simulink model "TEST1231"  (R2021a)
settings: Solver=VariableStepAuto  StartTime=0.0  StopTime=10.0  RelTol=1e-3
values from neighbouring files (symbols this model uses):
  phi0 = 0    [test.m]
  Rmin = 6    [Copy_of_main.m]    (also in parall.m)
  x0 = -8.5    [paralle.m]    (also in test.m = 9; verit.m = -3.7)
  y0 = -4    [paralle.m]    (also in test.m = 3; verit.m = -6.5)
libraries: dspstat3 x2
settings Model: Creator=6000022764  LastModifiedBy=6000022764

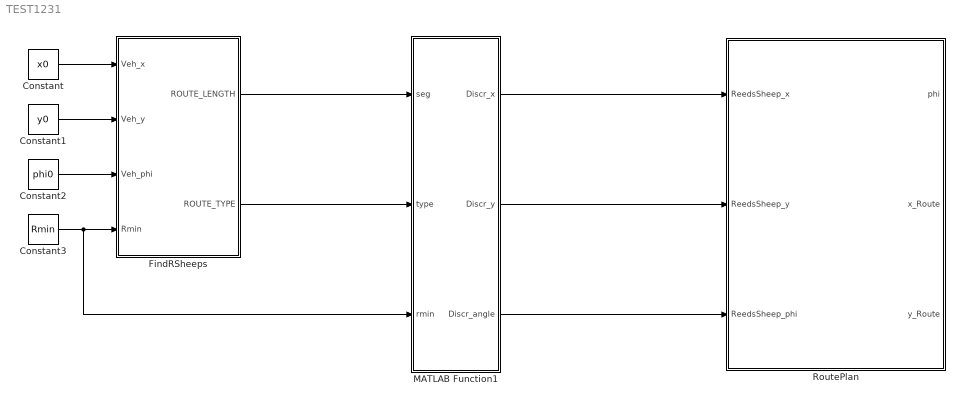
== system TEST1231 ==
  Constant : Constant  Value=x0
  Constant1 : Constant  Value=y0
  Constant2 : Constant  Value=phi0
  Constant3 : Constant  Value=Rmin
  FindRSheeps : Subsystem  Description=查找RS路径
      settings: AttributesFormatString=%<Description>
  MATLAB Function1 : MATLAB Function  TreatAsAtomicUnit=on
  RoutePlan : Subsystem  Description=B样条曲线
      settings: AttributesFormatString=%<Description>
  wires:
  Constant/1 -> FindRSheeps/1(Veh_x)
  Constant1/1 -> FindRSheeps/2(Veh_y)
  Constant3/1 -> MATLAB Function1/3(rmin), FindRSheeps/4(Rmin)
  Constant2/1 -> FindRSheeps/3(Veh_phi)
  FindRSheeps/1(ROUTE_LENGTH) -> MATLAB Function1/1(seg)
  FindRSheeps/2(ROUTE_TYPE) -> MATLAB Function1/2(type)
  MATLAB Function1/1(Discr_x) -> RoutePlan/1(ReedsSheep_x)
  MATLAB Function1/2(Discr_y) -> RoutePlan/2(ReedsSheep_y)
  MATLAB Function1/3(Discr_angle) -> RoutePlan/3(ReedsSheep_phi)

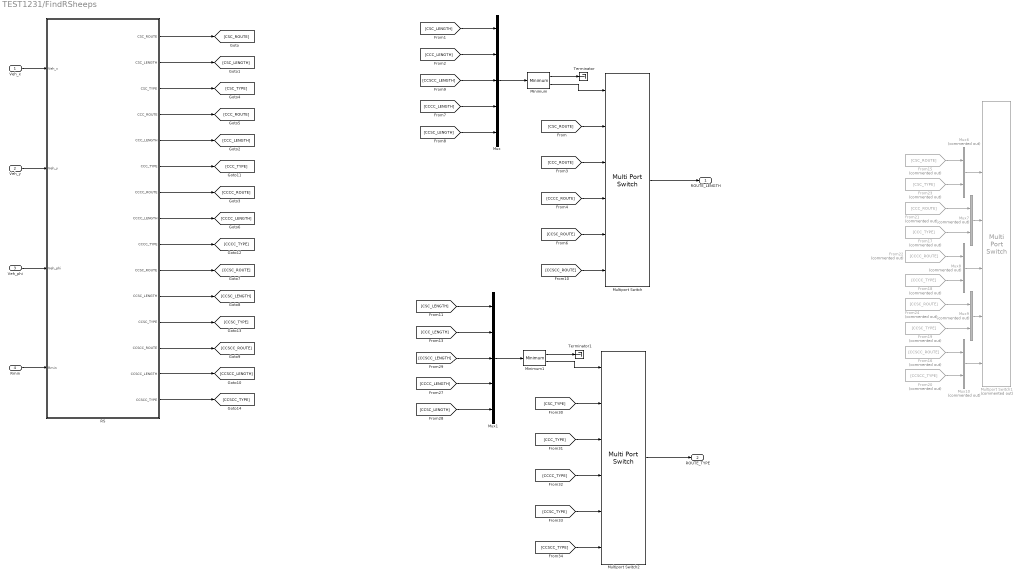
== system TEST1231/FindRSheeps ==
  Veh_x : Inport
  Veh_y : Inport  Port=2
  Veh_phi : Inport  Port=3
  Rmin : Inport  Port=4
  From15 : From  Commented=on  GotoTag=CSC_ROUTE
  From16 : From  Commented=on  GotoTag=CCSCC_ROUTE
  From17 : From  Commented=on  GotoTag=CCC_TYPE
  From18 : From  Commented=on  GotoTag=CCCC_TYPE
  From19 : From  Commented=on  GotoTag=CCSC_TYPE
  From20 : From  Commented=on  GotoTag=CCSCC_TYPE
  From21 : From  Commented=on  GotoTag=CCC_ROUTE
  From22 : From  Commented=on  GotoTag=CCCC_ROUTE
  From23 : From  Commented=on  GotoTag=CSC_TYPE
  From24 : From  Commented=on  GotoTag=CCSC_ROUTE
  Minimum : dspstat3/Minimum  operation=minimum  fcn=Value and Index  indexBase=One  operateOver=Each column  Dimension=1  InputProcessing=Columns as channels (frame based)  reset=None  roiEnable=off  roiType=Rectangles  roiPortion=Entire ROI  roiOutput=Individual statistics for each ROI  roiFlag=off  roundingMode=Floor  overflowMode=off
      settings: SourceProductBaseCode=DS
  Minimum1 : dspstat3/Minimum  operation=minimum  fcn=Value and Index  indexBase=One  operateOver=Each column  Dimension=1  InputProcessing=Columns as channels (frame based)  reset=None  roiEnable=off  roiType=Rectangles  roiPortion=Entire ROI  roiOutput=Individual statistics for each ROI  roiFlag=off  roundingMode=Floor  overflowMode=off
      settings: SourceProductBaseCode=DS
  Multiport Switch : MultiPortSwitch  Inputs=5
  Multiport Switch1 : MultiPortSwitch  Commented=on  Inputs=5
  Multiport Switch2 : MultiPortSwitch  Inputs=5
  Mux : Mux  Inputs=5
  Mux1 : Mux  Inputs=5
  Mux{6..10} (5 alike) : Mux  Commented=on  Inputs=2
  RS : Subsystem  Description=RS_word
      settings: AttributesFormatString=%<Description>
  Terminator : Terminator
  Terminator1 : Terminator
  ROUTE_LENGTH : Outport
  ROUTE_TYPE : Outport  Port=2
  wires:
  Minimum/1 -> Terminator/1
  [CCSCC_ROUTE] -> Multiport Switch/6
  [CCSC_ROUTE] -> Multiport Switch/5
  [CCC_ROUTE] -> Multiport Switch/3
  [CCCC_ROUTE] -> Multiport Switch/4
  RS/15(CCSCC_TYPE) -> [CCSCC_TYPE]
  RS/12(CCSC_TYPE) -> [CCSC_TYPE]
  RS/9(CCCC_TYPE) -> [CCCC_TYPE]
  RS/6(CCC_TYPE) -> [CCC_TYPE]
  [CSC_ROUTE] -> Multiport Switch/2
  RS/3(CSC_TYPE) -> [CSC_TYPE]
  Multiport Switch/1 -> ROUTE_LENGTH/1
  [CCSCC_LENGTH] -> Mux/3
  [CCSC_LENGTH] -> Mux/5
  [CCCC_LENGTH] -> Mux/4
  RS/14(CCSCC_LENGTH) -> [CCSCC_LENGTH]
  RS/13(CCSCC_ROUTE) -> [CCSCC_ROUTE]
  RS/11(CCSC_LENGTH) -> [CCSC_LENGTH]
  RS/10(CCSC_ROUTE) -> [CCSC_ROUTE]
  RS/8(CCCC_LENGTH) -> [CCCC_LENGTH]
  RS/7(CCCC_ROUTE) -> [CCCC_ROUTE]
  RS/5(CCC_LENGTH) -> [CCC_LENGTH]
  RS/4(CCC_ROUTE) -> [CCC_ROUTE]
  RS/2(CSC_LENGTH) -> [CSC_LENGTH]
  RS/1(CSC_ROUTE) -> [CSC_ROUTE]
  Rmin/1 -> RS/4(Rmin)
  Veh_phi/1 -> RS/3(Veh_phi)
  Veh_y/1 -> RS/2(Veh_y)
  Veh_x/1 -> RS/1(Veh_x)
  [CCC_LENGTH] -> Mux/2
  [CSC_LENGTH] -> Mux/1
  Mux/1 -> Minimum/1
  Minimum/2 -> Multiport Switch/1
  From15/1 -> Mux6/1
  From23/1 -> Mux6/2
  Mux6/1 -> Multiport Switch1/2
  From21/1 -> Mux7/1
  From17/1 -> Mux7/2
  From22/1 -> Mux8/1
  From18/1 -> Mux8/2
  From24/1 -> Mux9/1
  From19/1 -> Mux9/2
  From16/1 -> Mux10/1
  From20/1 -> Mux10/2
  Mux8/1 -> Multiport Switch1/4
  Mux7/1 -> Multiport Switch1/3
  Mux9/1 -> Multiport Switch1/5
  Mux10/1 -> Multiport Switch1/6
  Minimum1/2 -> Multiport Switch2/1
  Mux1/1 -> Minimum1/1
  [CSC_LENGTH] -> Mux1/1
  [CCC_LENGTH] -> Mux1/2
  [CCCC_LENGTH] -> Mux1/4
  [CCSC_LENGTH] -> Mux1/5
  [CCSCC_LENGTH] -> Mux1/3
  Multiport Switch2/1 -> ROUTE_TYPE/1
  [CSC_TYPE] -> Multiport Switch2/2
  [CCCC_TYPE] -> Multiport Switch2/4
  [CCC_TYPE] -> Multiport Switch2/3
  [CCSC_TYPE] -> Multiport Switch2/5
  [CCSCC_TYPE] -> Multiport Switch2/6
  Minimum1/1 -> Terminator1/1

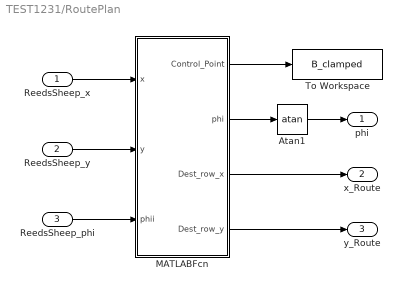
== system TEST1231/RoutePlan ==
  ReedsSheep_x : Inport
  ReedsSheep_y : Inport  Port=2
  ReedsSheep_phi : Inport  Port=3
  Atan1 : Trigonometry  Operator=atan
  MATLABFcn : MATLAB Function  Description=5次B样条开Clamped  TreatAsAtomicUnit=on
      settings: AttributesFormatString=%<Description>
  To Workspace : ToWorkspace  VariableName=B_clamped  SampleTime=-1
  phi : Outport  InitialOutput=0
  x_Route : Outport  Port=2  InitialOutput=9
  y_Route : Outport  Port=3  InitialOutput=3
  wires:
  MATLABFcn/1(Control_Point) -> To Workspace/1
  MATLABFcn/2(phi) -> Atan1/1
  Atan1/1 -> phi/1
  MATLABFcn/3(Dest_row_x) -> x_Route/1
  MATLABFcn/4(Dest_row_y) -> y_Route/1
  ReedsSheep_x/1 -> MATLABFcn/1(x)
  ReedsSheep_y/1 -> MATLABFcn/2(y)
  ReedsSheep_phi/1 -> MATLABFcn/3(phii)

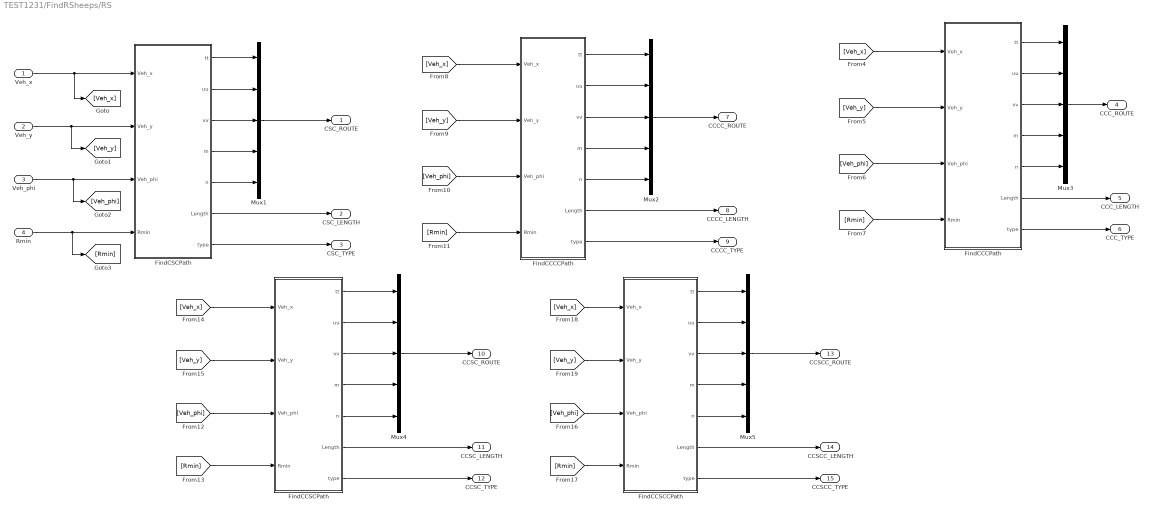
== system TEST1231/FindRSheeps/RS ==
  Veh_x : Inport
  Veh_y : Inport  Port=2
  Veh_phi : Inport  Port=3
  Rmin : Inport  Port=4
  FindCCCCPath : Stateflow chart  Description=查找CCCC路径  TreatAsAtomicUnit=on
      settings: AttributesFormatString=%<Description>  RTWSystemCode=Inline
  FindCCCPath : Stateflow chart  Description=查找CCC路径  TreatAsAtomicUnit=on
      settings: AttributesFormatString=%<Description>  RTWSystemCode=Inline
  FindCCSCCPath : Stateflow chart  Description=查找CCSCC路径  TreatAsAtomicUnit=on
      settings: AttributesFormatString=%<Description>  RTWSystemCode=Inline
  FindCCSCPath : Stateflow chart  Description=查找CCSC路径  TreatAsAtomicUnit=on
      settings: AttributesFormatString=%<Description>  RTWSystemCode=Inline
  FindCSCPath : Stateflow chart  Description=查找CSC路径  TreatAsAtomicUnit=on
      settings: AttributesFormatString=%<Description>  RTWSystemCode=Inline
  Mux{1..5} (5 alike) : Mux  Inputs=5
  CSC_ROUTE : Outport
  CSC_LENGTH : Outport  Port=2
  CSC_TYPE : Outport  Port=3
  CCC_ROUTE : Outport  Port=4
  CCC_LENGTH : Outport  Port=5
  CCC_TYPE : Outport  Port=6
  CCCC_ROUTE : Outport  Port=7
  CCCC_LENGTH : Outport  Port=8
  CCCC_TYPE : Outport  Port=9
  CCSC_ROUTE : Outport  Port=10
  CCSC_LENGTH : Outport  Port=11
  CCSC_TYPE : Outport  Port=12
  CCSCC_ROUTE : Outport  Port=13
  CCSCC_LENGTH : Outport  Port=14
  CCSCC_TYPE : Outport  Port=15
  wires:
  FindCCSCCPath/7(type) -> CCSCC_TYPE/1
  FindCCSCPath/7(type) -> CCSC_TYPE/1
  FindCCCCPath/7(type) -> CCCC_TYPE/1
  FindCCCPath/7(type) -> CCC_TYPE/1
  FindCSCPath/7(type) -> CSC_TYPE/1
  [Rmin] -> FindCCSCCPath/4(Rmin)
  [Veh_phi] -> FindCCSCCPath/3(Veh_phi)
  [Veh_y] -> FindCCSCCPath/2(Veh_y)
  [Veh_x] -> FindCCSCCPath/1(Veh_x)
  FindCCSCCPath/1(tt) -> Mux5/1
  FindCCSCCPath/5(n) -> Mux5/5
  FindCCSCCPath/3(vv) -> Mux5/3
  FindCCSCCPath/2(uu) -> Mux5/2
  FindCCSCCPath/4(m) -> Mux5/4
  FindCCSCCPath/6(Length) -> CCSCC_LENGTH/1
  Mux5/1 -> CCSCC_ROUTE/1
  [Rmin] -> FindCCSCPath/4(Rmin)
  [Veh_phi] -> FindCCSCPath/3(Veh_phi)
  [Veh_y] -> FindCCSCPath/2(Veh_y)
  [Veh_x] -> FindCCSCPath/1(Veh_x)
  FindCCSCPath/1(tt) -> Mux4/1
  FindCCSCPath/5(n) -> Mux4/5
  FindCCSCPath/3(vv) -> Mux4/3
  FindCCSCPath/2(uu) -> Mux4/2
  FindCCSCPath/4(m) -> Mux4/4
  FindCCSCPath/6(Length) -> CCSC_LENGTH/1
  Mux4/1 -> CCSC_ROUTE/1
  Mux2/1 -> CCCC_ROUTE/1
  FindCCCCPath/6(Length) -> CCCC_LENGTH/1
  FindCCCCPath/4(m) -> Mux2/4
  FindCCCCPath/2(uu) -> Mux2/2
  FindCCCCPath/3(vv) -> Mux2/3
  FindCCCCPath/5(n) -> Mux2/5
  FindCCCCPath/1(tt) -> Mux2/1
  [Veh_x] -> FindCCCCPath/1(Veh_x)
  [Veh_y] -> FindCCCCPath/2(Veh_y)
  [Veh_phi] -> FindCCCCPath/3(Veh_phi)
  [Rmin] -> FindCCCCPath/4(Rmin)
  [Veh_x] -> FindCCCPath/1(Veh_x)
  [Veh_y] -> FindCCCPath/2(Veh_y)
  [Veh_phi] -> FindCCCPath/3(Veh_phi)
  [Rmin] -> FindCCCPath/4(Rmin)
  Rmin/1 -> [Rmin], FindCSCPath/4(Rmin)
  Veh_y/1 -> [Veh_y], FindCSCPath/2(Veh_y)
  Veh_x/1 -> FindCSCPath/1(Veh_x), [Veh_x]
  Veh_phi/1 -> [Veh_phi], FindCSCPath/3(Veh_phi)
  FindCCCPath/5(n) -> Mux3/5
  FindCCCPath/3(vv) -> Mux3/3
  FindCCCPath/4(m) -> Mux3/4
  FindCCCPath/2(uu) -> Mux3/2
  FindCCCPath/1(tt) -> Mux3/1
  FindCCCPath/6(Length) -> CCC_LENGTH/1
  Mux3/1 -> CCC_ROUTE/1
  FindCSCPath/1(tt) -> Mux1/1
  FindCSCPath/5(n) -> Mux1/5
  FindCSCPath/3(vv) -> Mux1/3
  FindCSCPath/2(uu) -> Mux1/2
  FindCSCPath/4(m) -> Mux1/4
  FindCSCPath/6(Length) -> CSC_LENGTH/1
  Mux1/1 -> CSC_ROUTE/1

== stateflow chart TEST1231/FindRSheeps/RS/FindCSCPath ==
  state Begin
    entry:
    rmin = Rmin;
    x_F = Veh_x/rmin;
    y_F = Veh_y/rmin;
    phi_F = Veh_phi;
    [isok,tt,uu,vv] = LpSpLp(x_F,y_F,phi_F);
    type = 'NNNNN';Length=1000;
  state RmSmLm
    entry:
    [isok,tt,uu,vv] = LpSpRp(-x_F,-y_F,phi_F);
    Length = 1000;
    m = 0;
    n = 0;
  state LmSmRm
    entry:
    [isok,tt,uu,vv] = LpSpRp(-x_F,y_F,-phi_F);
  state RpSpLp
    entry:
    [isok,tt,uu,vv] = LpSpRp(x_F,-y_F,-phi_F);
  state stand7
    Length = 1000;
    tt=0;vv=0;uu=0;
    n = 0;m= 0;
    type = 'NNNNN';
  state LpSpRp_main
    entry:
    [isok,tt,uu,vv] = LpSpRp(x_F,y_F,phi_F);
  state LmSmLm
    entry:
    [isok,tt,uu,vv] = LpSpLp(-x_F,y_F,-phi_F);
  state RpSpRp
    entry:
    [isok,tt,uu,vv] = LpSpLp(x_F,-y_F,-phi_F);
  state RmSmRm
    entry:
    [isok,tt,uu,vv] = LpSpLp(-x_F,-y_F,phi_F);
  state LpSpLp_ok
    Length = abs(tt) +abs(uu)+abs(vv);
    m = 0;
    n = 0;
    type = 'LSLNN';
  state LpSpLp_ok1
    Length = abs(tt) +abs(uu)+abs(vv);
    m = 0;
    n = 0;
    type = 'LSLNN';
  state RpSpRp_ok
    Length = abs(tt) +abs(uu)+abs(vv);
    m = 0;
    n = 0;
    type = 'RSRNN';
  state RmSmRm_ok
    Length = abs(tt) +abs(uu)+abs(vv);
    m = 0;
    n = 0;
    type = 'RSRNN';
  state LpSpRp_ok
    Length = abs(tt) +abs(uu)+abs(vv);
    m = 0;
    n = 0;
    type = 'LSRNN';
  state LmSmRm_ok
    Length = abs(tt) +abs(uu)+abs(vv);
    m = 0;
    n = 0;
    type = 'LSRNN';
  state RpSpLp_ok
    Length = abs(tt) +abs(uu)+abs(vv);
    m = 0;
    n = 0;
    type = 'RSLNN';
  state RmSmLm_ok
    Length = abs(tt) +abs(uu)+abs(vv);
    m = 0;tt=-tt;uu=-uu;vv=-vv;
    n = 0;
    type = 'RSLNN';
  state stand1
  state stand2
  state stand3
  state stand4
  state stand5
  state stand6
  state stand
  state stand8
  (default) -> Begin
  RmSmLm -> stand7 [order 2] : [isok==0]
  LmSmRm -> RpSpLp [order 2] : [isok == 0]
  RpSpLp -> RmSmLm [order 2] : [isok == 0]
  LmSmLm -> RpSpRp [order 2] : [isok == 0]
  Begin -> LmSmLm [order 2] : [isok == 0]
  RpSpRp -> RmSmRm [order 1] : [isok == 0]
  LpSpRp_main -> LmSmRm [order 2] : [isok ==0]
  RmSmRm -> LpSpRp_main [order 1] : [isok == 0]
  LpSpRp_main -> LpSpRp_ok [order 1] : [isok ==1]
  Begin -> LpSpLp_ok [order 1] : [isok == 1]
  LmSmLm -> LpSpLp_ok1 [order 1] : [isok == 1]
  RpSpRp -> RpSpRp_ok [order 2] : [isok == 1]
  RmSmRm -> RmSmRm_ok [order 2] : [isok ==1]
  RpSpLp -> RpSpLp_ok [order 1] : [isok ==1]
  RmSmLm -> RmSmLm_ok [order 1] : [isok ==1]
  LmSmRm -> LmSmRm_ok [order 1] : [isok ==1]
  LpSpLp_ok -> stand
  LpSpLp_ok1 -> stand1
  RpSpRp_ok -> stand2
  RmSmRm_ok -> stand3
  LpSpRp_ok -> stand4
  LmSmRm_ok -> stand5
  RpSpLp_ok -> stand6
  RmSmLm_ok -> stand8
  data: x function_input double; y function_input double; phi function_input double; isok function_output double; t function_output double; u function_output double; v function_output double; x function_input double; v function_output double; x function_input double; y function_input double; phi function_input double; isok function_output double; t function_output double; u function_output double; v function_output double; Veh_x input double; Veh_y input double; Veh_phi input double; Rmin input double; tt output double; uu output double; vv output double; m output double; n output double; Length output double; type output string; isok local double; phi_F local double; rmin local double; x_F local double; y_F local double
  function [isok, t,u,v] = LpSpRp(x,y,phi):
    | function [isok, t,u,v] = LpSpRp(x,y,phi)
    |     [t1,u1] = cart2pol(x+sin(phi),y-1-cos(phi));
    |     if u1^2 >= 4
    |         u = sqrt(u1^2-4);
    |         theta = atan2(2,u);
    |         t = mod2pi(t1+theta);
    |         v = mod2pi(t-phi);
    |         if t >= 0 && v >= 0 % 符号代表前进和后退
    |             isok = 1;
    |             return
    |         end
    |     end
    |     isok = 0;
    |     t = 0;
    |     u = 0;
    |     v = 0;
    | end
  function v = mod2pi(x):
    | function v = mod2pi(x)
    |     v = rem(x,2*pi);
    |     if v < -pi
    |         v = v+2*pi;
    |     elseif v > pi
    |         v = v-2*pi;
    |     end
    | end
  function [isok,t,u,v] = LpSpLp(x,y,phi):
    | function [isok,t,u,v] = LpSpLp(x,y,phi)
    |     [t,u] = cart2pol(x-sin(phi),y-1+cos(phi));
    |     if t >= 0
    |         v = mod2pi(phi-t);
    |         if v >= 0
    |             isok = 1;
    |             return
    |         end
    |     end
    |     isok = 0;
    |     t = 0;
    |     u = 0;
    |     v = 0;
    | end

== stateflow chart TEST1231/FindRSheeps/RS/FindCCCCPath ==
  state Begin
    entry:
    rmin = Rmin;
    x_F = Veh_x/rmin;
    y_F = Veh_y/rmin;
    phi_F = Veh_phi;
    [isok,tt,uu,vv] = LpRupLumRm(x_F,y_F,phi_F);
    type = 'NNNNN';Length=1000;
  state LmRumLupRp
    entry:
    [isok,tt,uu,vv] = LpRupLumRm(-x_F,y_F,-phi_F);
  state RpLupRumLm
    entry:
    [isok,tt,uu,vv] = LpRupLumRm(x_F,-y_F,-phi_F);
  state RmLupRupLm
    entry:
    [isok,tt,uu,vv] = LpRumLumRp(-x_F,-y_F,phi_F);
    Length = 1000;
    m=0;n=0;
  state LmRupLupRm
    entry:
    [isok,tt,uu,vv] = LpRumLumRp(-x_F,y_F,-phi_F);
  state RpLumRumLp
    entry:
    [isok,tt,uu,vv] = LpRumLumRp(x_F,-y_F,-phi_F);
  state LpRumLumRp_main
    entry:
    [isok,tt,uu,vv] = LpRumLumRp(x_F,y_F,phi_F);
  state stand7
    Length = 1000;
    tt=0;vv=0;uu=0;
    n = 0;m= 0;
    type = 'NNNNN';
  state RmLumRupLp
    entry:
    [isok,tt,uu,vv] = LpRupLumRm(-x_F,-y_F,phi_F);
  state LpRupLumRm_ok
    Length = abs(tt) +2*abs(uu)+abs(vv);
    m = vv;
    vv=-uu;
    n = 0;
    type = 'LRLRN';
  state LmRumLupRp_ok
    Length = abs(tt) +2*abs(uu)+abs(vv);
    tt=-tt;vv=uu;uu=-uu;
    m = -vv;
    n = 0;
    type = 'LRLRN';
  state RpLupRumLm_ok
    Length = abs(tt) +2*abs(uu)+abs(vv);
    m = vv;
    vv=-uu;
    n = 0;
    type = 'RLRLN';
  state RmLumRupLp_ok
    Length = abs(tt) +2*abs(uu)+abs(vv);
    m = -vv;tt=-tt;vv=uu;uu=-uu;
    n = 0;
    type = 'RLRLN';
  state LmRupLupRm_ok
    Length = abs(tt) +2*abs(uu)+abs(vv);
    m = -vv;tt=-tt;vv=-uu;uu=-uu;
    n = 0;
    type = 'LRLRN';
  state RpLumRumLp_ok
    Length = abs(tt) +2*abs(uu)+abs(vv);
    m = vv;vv=uu;
    n = 0;
    type = 'RLRLN';
  state RmLupRupLm_ok
    Length = abs(tt) +abs(uu)+abs(vv);
    m = -vv;tt=-tt;vv=-uu;uu=-uu;
    n = 0;
    type = 'RLRLN';
  state LpRumLumRp_ok
    Length = abs(tt) +2*abs(uu)+abs(vv);
    m = vv;vv=uu;
    n = 0;
    type = 'LRLRN';
  state stand
  state stand2
  state stand1
  state stand3
  state stand4
  state stand5
  state stand6
  (default) -> Begin
  LmRumLupRp -> RpLupRumLm [order 2] : [isok == 0]
  Begin -> LmRumLupRp [order 2] : [isok == 0]
  RmLupRupLm -> stand7 [order 2] : [isok==0]
  RpLupRumLm -> RmLumRupLp [order 1] : [isok == 0]
  RmLumRupLp -> LpRumLumRp_main [order 1] : [isok == 0]
  LmRupLupRm -> RpLumRumLp [order 2] : [isok == 0]
  LpRumLumRp_main -> LmRupLupRm [order 2] : [isok ==0]
  RpLumRumLp -> RmLupRupLm [order 2] : [isok == 0]
  Begin -> LpRupLumRm_ok [order 1] : [isok == 1]
  LmRumLupRp -> LmRumLupRp_ok [order 1] : [isok == 1]
  RpLupRumLm -> RpLupRumLm_ok [order 2] : [isok == 1]
  RmLumRupLp -> RmLumRupLp_ok [order 2] : [isok ==1]
  LpRumLumRp_main -> LpRumLumRp_ok [order 1] : [isok ==1]
  LmRupLupRm -> LmRupLupRm_ok [order 1] : [isok ==1]
  RpLumRumLp -> RpLumRumLp_ok [order 1] : [isok ==1]
  RmLupRupLm -> RmLupRupLm_ok [order 1] : [isok ==1]
  RmLumRupLp_ok -> stand3
  LmRupLupRm_ok -> stand5
  LpRupLumRm_ok -> stand
  RpLupRumLm_ok -> stand2
  RpLumRumLp_ok -> stand6
  LpRumLumRp_ok -> stand4
  LmRumLupRp_ok -> stand1
  data: x function_input double; v function_output double; x function_input double; y function_input double; phi function_input double; isok function_output double; t function_output double; u function_output double; v function_output double; u function_input double; v function_input double; xi function_input double; eta function_input double; phi function_input double; tau function_output double; omega function_output double; x function_input double; y function_input double; phi function_input double; isok function_output double; t function_output double; u function_output double; v function_output double; Veh_x input double; Veh_y input double; Veh_phi input double; Rmin input double; tt output double; uu output double; vv output double; m output double; n output double; Length output double; type output string; isok local double; phi_F local double; rmin local double; x_F local double; y_F local double
  function v = mod2pi(x):
    | function v = mod2pi(x)
    |     v = rem(x,2*pi);
    |     if v < -pi
    |         v = v+2*pi;
    |     elseif v > pi
    |         v = v-2*pi;
    |     end
    | end
  function [isok,t,u,v] = LpRupLumRm(x,y,phi):
    | function [isok,t,u,v] = LpRupLumRm(x,y,phi)
    |     xi = x+sin(phi);
    |     eta = y-1-cos(phi);
    |     rho = (2+sqrt(xi^2+eta^2))/4;
    |     if rho <= 1
    |         u = acos(rho);
    |         [t,v] = tauOmega(u,-u,xi,eta,phi);
    |         if t >= 0 && v <= 0
    |             isok = 1;
    |             return
    |         end
    |     end
    |     isok = 0;
    |     t = 0;
    |     u = 0;
    |     v = 0;
    | end
  function [tau,omega] = tauOmega(u,v,xi,eta,phi):
    | function [tau,omega] = tauOmega(u,v,xi,eta,phi)
    |     delta = mod2pi(u-v);
    |     A = sin(u)-sin(delta);
    |     B = cos(u)-cos(delta)-1;
    |     t1 = atan2(eta*A-xi*B,xi*A+eta*B);
    |     t2 = 2*(cos(delta)-2*cos(v)-2*cos(u))+3;
    |     if t2 < 0
    |         tau = mod2pi(t1+pi);
    |     else
    |         tau = mod2pi(t1);
    |     end
    |     omega = mod2pi(tau-u+v-phi);
    | end
  function [isok,t,u,v] = LpRumLumRp(x,y,phi):
    | function [isok,t,u,v] = LpRumLumRp(x,y,phi)
    |     xi = x+sin(phi);
    |     eta = y-1-cos(phi);
    |     rho = (20-xi^2-eta^2)/16;
    |     if rho >= 0 && rho <= 1
    |         u = -acos(rho);
    |         if u >= -pi/2
    |             [t,v] = tauOmega(u,u,xi,eta,phi);
    |             if t >=0 && v >=0
    |                 isok = 1;
    |                 return
    |             end
    |         end
    |     end
    |     isok = 0;
    |     t = 0;
    |     u = 0;
    |     v = 0;
    | end

== matlab function TEST1231/MATLAB Function1 ==
  data: seg input; Discr_x output; Discr_y output; Discr_angle output; type input; rmin input
function [Discr_x,Discr_y,Discr_angle] = fcn(seg,type,rmin)
% seg = [t,u,v,m,n];
type = char(type);
x=zeros(500,1);y=zeros(500,1);angle=zeros(500,1);
Discr_x=zeros(15,1);
Discr_y=zeros(15,1);Discr_angle=zeros(15,1);
pvec=[0,0,0];
for i = 1:5
    if type(i) == 'S'
        theta = pvec(3);
        dl = rmin*seg(i);
        dvec = [dl*cos(theta), dl*sin(theta), 0];
        dx = pvec(1)+linspace(0,dvec(1));
        dy = pvec(2)+linspace(0,dvec(2));
        Routephi = theta*linspace(1,1);
        x((1+100*(i-1)):100*i) = dx;
        y((1+100*(i-1)):100*i) = dy;
        angle((1+100*(i-1)):100*i) = Routephi;
        Discr_x((1+5*(i-1)):5*i) = dx(1:23:end);
        Discr_y((1+5*(i-1)):5*i) = dy(1:23:end);
        Discr_angle((1+5*(i-1)):5*i) = Routephi(1:23:end);
        pvec = pvec+dvec;
    elseif type(i) == 'L'
        theta = pvec(3);
        dtheta = seg(i);
        cenx = pvec(1)-rmin*sin(theta);
        ceny = pvec(2)+rmin*cos(theta);
        t = theta-pi/2+linspace(0,dtheta);
        Routephi = theta + linspace(0,dtheta);
        dx = cenx+rmin*cos(t);
        dy = ceny+rmin*sin(t);
        x((1+100*(i-1)):100*i) = dx;
        y((1+100*(i-1)):100*i) = dy;
        angle((1+100*(i-1)):100*i) = Routephi;
        Discr_x((1+5*(i-1)):5*i) = dx(1:23:end);
        Discr_y((1+5*(i-1)):5*i) = dy(1:23:end);
        Discr_angle((1+5*(i-1)):5*i) = Routephi(1:23:end);
        theta = theta+dtheta;
        pvec = [dx(end),dy(end),theta];
    elseif type(i) == 'R'
        theta = pvec(3);
        dtheta = -seg(i);
        cenx = pvec(1)+rmin*sin(theta);
        ceny = pvec(2)-rmin*cos(theta);
        t = theta+pi/2+linspace(0,dtheta);
        Routephi  = theta + linspace(0,dtheta);
        dx = cenx+rmin*cos(t);
        dy = ceny+rmin*sin(t);
        x((1+100*(i-1)):100*i) = dx;
        y((1+100*(i-1)):100*i) = dy;
        angle((1+100*(i-1)):100*i) = Routephi;
        Discr_x((1+5*(i-1)):5*i) = dx(1:23:end);
        Discr_y((1+5*(i-1)):5*i) = dy(1:23:end);
        Discr_angle((1+5*(i-1)):5*i) = Routephi(1:23:end);
        theta = theta+dtheta;
        pvec = [dx(end),dy(end),theta];
    else
        x((1+100*(i-1)):100*i) = nan;
        y((1+100*(i-1)):100*i) = nan;
        angle((1+100*(i-1)):100*i) = nan;
    end
%     nonan_x = x(~isnan(x));
%     nonan_y = y(~isnan(y));
%     nonan_angle = angle(~isnan(angle));
%     Discr_x = x(1:20:end);
%     Discr_y = y(1:20:end);
%     Discr_angle = angle(1:10:end);
end

== matlab function TEST1231/RoutePlan/MATLABFcn ==
  data: Control_Point output; x input; phi output; Dest_row_x output; Dest_row_y output; y input; phii input
function [Control_Point,phi,Dest_row_x,Dest_row_y] = fcn(x,y,phii)
% n,线条控制点数；k，阶次数
% clear all;
n =15; k =5;
% n =7; k =5;
P_dest = zeros(2,n);
P_dest(1,:) = x;
P_dest(2,:) = y;
% NodeVector = linspace(0,1,n+k+1); % 从0到1，设置均匀B样条节点区间；
% NodeVector = [0,0,0,0,0,0,0.2,0.4,0.6,0.8,1,1,1,1,1,1];
% NodeVector = [0,0,0,0,0,0,0.5,1,1,1,1,1,1];
% NodeVector = [0,0,0,0,0,0,0.1,0.2,0.3,0.4,0.5,0.6,0.7,0.8,0.9,1,1,1,1,1,1];
NodeVector = [0,0,0,0,0,0,1,2,3,4,5,6,7,8,9,10,10,10,10,10,10];
% NodeVector = [0,0,0,0,0,0,0.05,0.1,0.15,0.2,0.25,0.3,0.35,0.4,0.45,0.5,0.55,0.6,0.65,0.7,0.75,0.8,0.85,0.9,0.95,1,1,1,1,1,1];
% 当起始点和终止点的重复度为最高次数加1是，开B样条变为Clamped B样条，当起始点和终止点重合且重复度为p+1时为闭B样条曲线。
Nik = zeros(n+k, k+1);
plot(P_dest(1, 1:n), P_dest(2, 1:n),...
    'o','LineWidth',1,...
    'MarkerEdgeColor','k',...
    'MarkerFaceColor','g',...
    'MarkerSize',6);%hold on;
line(P_dest(1, 1:n), P_dest(2, 1:n));hold on;
% axis([-2,10,-2,10]);
umin =0;umax = 10;delta_u = 0.02;
Num = floor((umax-umin)/delta_u)+1;
Dest = zeros(2,Num);
Control_Point = zeros(Num,3);
Dest_row_x = zeros(Num,1);
Dest_row_y = zeros(Num,1);
m=1;
phi = zeros(Num,1);
N_i_5 = zeros(n,1);
for u = umin : delta_u : umax
    for i5 = 1:n
        for i4 = i5:i5+1
            for i3 = i5:i5+2
                for i2 = i5:i5+3
                    for i1 = i5:i5+4
                        for i = i5:i5+5
                            if (u >= NodeVector(i)) && (u < NodeVector(i+1))
                                Nik(i,1) = 1.0;
                            else
                                Nik(i,1) = 0.0;
                            end
                        end
                        Length1 = NodeVector(i1+1) - NodeVector(i1);
                        Length2 = NodeVector(i1+2) - NodeVector(i1+1);      % 支撑区间的长度
                        if Length1 == 0.0       % 规定0/0 = 0
                            Length1 = 1.0;
                        end
                        if Length2 == 0.0
                            Length2 = 1.0;
                        end
                        Nik(i1,2) = (u - NodeVector(i1)) / Length1 * Nik(i1,1) ...
                            + (NodeVector(i1+2) - u) / Length2 * Nik(i1+1,1);
                    end
                    Length1 = NodeVector(i2+2) - NodeVector(i2);
                    Length2 = NodeVector(i2+3) - NodeVector(i2+1);      % 支撑区间的长度
                    if Length1 == 0.0       % 规定0/0 = 0
                        Length1 = 1.0;
                    end
                    if Length2 == 0.0
                        Length2 = 1.0;
                    end
                    Nik(i2,3) = (u - NodeVector(i2)) / Length1 * Nik(i2,2) ...
                        + (NodeVector(i2+3) - u) / Length2 * Nik(i2+1,2);
                end
                Length1 = NodeVector(i3+3) - NodeVector(i3);
                Length2 = NodeVector(i3+4) - NodeVector(i3+1);      % 支撑区间的长度
                if Length1 == 0.0       % 规定0/0 = 0
                    Length1 = 1.0;
                end
                if Length2 == 0.0
                    Length2 = 1.0;
                end
                Nik(i3,4) = (u - NodeVector(i3)) / Length1 * Nik(i3,3) ...
                    + (NodeVector(i3+4) - u) / Length2 * Nik(i3+1,3);
            end
            Length1 = NodeVector(i4+4) - NodeVector(i4);
            Length2 = NodeVector(i4+5) - NodeVector(i4+1);      % 支撑区间的长度
            if Length1 == 0.0       % 规定0/0 = 0
                Length1 = 1.0;
            end
            if Length2 == 0.0
                Length2 = 1.0;
            end
            Nik(i4,5) = (u - NodeVector(i4)) / Length1 * Nik(i4,4) ...
                + (NodeVector(i4+5) - u) / Length2 * Nik(i4+1,4);
        end
        Length1 = NodeVector(i5+5) - NodeVector(i5);
        Length2 = NodeVector(i5+6) - NodeVector(i5+1);      % 支撑区间的长度
        if Length1 == 0.0       % 规定0/0 = 0
            Length1 = 1.0;
        end
        if Length2 == 0.0
            Length2 = 1.0;
        end
        Nik(i5,6) = (u - NodeVector(i5)) / Length1 * Nik(i5,5) ...
            + (NodeVector(i5+6) - u) / Length2 * Nik(i5+1,5);
        N_i_5(i5,1) = Nik(i5,6);
    end
    p_u = P_dest * N_i_5;
    Dest(:,m) = p_u;
    Dest_row_x(m,1) = p_u(1,1);
    Dest_row_y(m,1) = p_u(2,1);
    if m>1 && min(Dest(:,m))>0
        phi(m,1) = (Dest(2,m-1) - Dest(2,m))/(Dest(1,m-1) - Dest(1,m));
    end
    Control_Point(m,:) = [Dest(:,m)' phi(m,1) ];
    m = m+1;
    
end
% phi(1,1) = phii(1,1);
phi(end,1) = phii(1,end);
Dest_row_x(end) = P_dest(1,end);
Dest_row_y(end) = P_dest(2,end);
Dest_row_x = flipud(Dest_row_x);
Dest_row_y = flipud(Dest_row_y);
phi = flipud(phi);
plot(Dest_row_x, Dest_row_y,'LineWidth',1,'Color','r');hold off;

== stateflow chart TEST1231/FindRSheeps/RS/FindCCCPath ==
  state Begin
    entry:
    rmin = Rmin;
    x_F = Veh_x/rmin;
    y_F = Veh_y/rmin;
    phi_F = Veh_phi;Length=1000;
    [isok,tt,uu,vv] = LpRmL(x_F,y_F,phi_F);
    type = 'NNNNN';
  state LRmLp
    entry:
    xb = x_F*cos(phi_F)+y_F*sin(phi_F);
    yb = x_F*sin(phi_F)-y_F*cos(phi_F);
    [isok,tt,uu,vv] = LpRmL(xb,yb,phi_F);
  state LRpLm
    entry:
    [isok,tt,uu,vv] = LpRmL(-xb,yb,-phi_F);
  state RLmRp
    entry:
    [isok,tt,uu,vv] = LpRmL(xb,-yb,-phi_F);
  state RLpRm_N_ok
    Length = 1000;
    tt=0;vv=0;uu=0;
    n = 0;m= 0;
    type = 'NNNNN';
  state RLpRm
    entry:
    [isok,tt,uu,vv] = LpRmL(-xb,-yb,phi_F);
  state LmRpL
    entry:
    [isok,tt,uu,vv] = LpRmL(-x_F,y_F,-phi_F);
  state RpLmR
    entry:
    [isok,tt,uu,vv] = LpRmL(x_F,-y_F,-phi_F);
  state RmLpR
    entry:
    [isok,tt,uu,vv] = LpRmL(-x_F,-y_F,phi_F);
  state LpRmL_ok
    Length = abs(tt) +abs(uu)+abs(vv);
    m = 0;
    n = 0;
    type = 'LRLNN';
  state LmRpL_ok
    Length = abs(tt) +abs(uu)+abs(vv);
    tt=-tt;uu=-uu;vv=-vv;
    m = 0;
    n = 0;
    type = 'LRLNN';
  state RpLmR_ok
    Length = abs(tt) +abs(uu)+abs(vv);
    m = 0;
    n = 0;
    type = 'RLRNN';
  state RmLpR_ok
    Length = abs(tt) +abs(uu)+abs(vv);
    tt=-tt;uu=-uu;vv=-vv;
    m = 0;
    n = 0;
    type = 'RLRNN';
  state LRmLp_ok
    Length = abs(tt) +abs(uu)+abs(vv);
    m = tt;tt=vv;vv=uu;uu=m;
    n = 0;m=0;
    type = 'LRLNN';
  state LRpLm_ok
    Length = abs(tt) +abs(uu)+abs(vv);
    m = tt;tt=-vv;vv=-uu;uu=-m;
    n = 0;m= 0;
    type = 'LRLNN';
  state RLmRp_ok
    Length = abs(tt) +abs(uu)+abs(vv);
    m = tt;tt=vv;vv=uu;uu=m;
    n = 0;m=0;
    type = 'RLRNN';
  state RLpRm_ok
    Length = abs(tt) +abs(uu)+abs(vv);
    m = tt;tt=-vv;vv=-uu;uu=-m;
    n = 0;m= 0;
    type = 'RLRNN';
  state stand2
  state stand1
  state stand
  state stand3
  state stand4
  state stand6
  state stand7
  state stand5
  (default) -> Begin
  LRpLm -> RLmRp [order 2] : [isok == 0]
  RLmRp -> RLpRm [order 2] : [isok == 0]
  LRmLp -> LRpLm [order 2] : [isok ==0]
  RLpRm -> RLpRm_N_ok [order 2] : [isok==0]
  LmRpL -> RpLmR [order 2] : [isok == 0]
  Begin -> LmRpL [order 2] : [isok == 0]
  RpLmR -> RmLpR [order 1] : [isok == 0]
  RmLpR -> LRmLp [order 1] : [isok == 0]
  Begin -> LpRmL_ok [order 1] : [isok == 1]
  LmRpL -> LmRpL_ok [order 1] : [isok == 1]
  RpLmR -> RpLmR_ok [order 2] : [isok == 1]
  RmLpR -> RmLpR_ok [order 2] : [isok ==1]
  LRpLm -> LRpLm_ok [order 1] : [isok ==1]
  RLmRp -> RLmRp_ok [order 1] : [isok ==1]
  RLpRm -> RLpRm_ok [order 1] : [isok ==1]
  LRmLp -> LRmLp_ok [order 1] : [isok ==1]
  LRmLp_ok -> stand6
  LpRmL_ok -> stand1
  RpLmR_ok -> stand2
  LRpLm_ok -> stand7
  RLmRp_ok -> stand4
  RLpRm_ok -> stand5
  LmRpL_ok -> stand
  RmLpR_ok -> stand3
  data: x function_input double; v function_output double; x function_input double; y function_input double; phi function_input double; isok function_output double; t function_output double; u function_output double; v function_output double; Veh_x input double; Veh_y input double; Veh_phi input double; Rmin input double; tt output double; uu output double; vv output double; m output double; n output double; Length output double; type output string; isok local double; phi_F local double; rmin local double; x_F local double; xb local double; y_F local double; yb local double
  function v = mod2pi(x):
    | function v = mod2pi(x)
    |     v = rem(x,2*pi);
    |     if v < -pi
    |         v = v+2*pi;
    |     elseif v > pi
    |         v = v-2*pi;
    |     end
    | end
  function [isok,t,u,v] = LpRmL(x,y,phi):
    | function [isok,t,u,v] = LpRmL(x,y,phi)
    |     xi = x-sin(phi);
    |     eta = y-1+cos(phi);
    |     [theta,u1] = cart2pol(xi,eta);
    |     if u1 <= 4
    |         u = -2*asin(u1/4);
    |         t = mod2pi(theta+u/2+pi);
    |         v = mod2pi(phi-t+u);
    |         if t >= 0 && u <= 0
    |             isok = 1;
    |             return
    |         end
    |     end
    |     isok = 0;
    |     t = 0;
    |     u = 0;
    |     v = 0;
    | end

== stateflow chart TEST1231/FindRSheeps/RS/FindCCSCPath ==
  state Begin
    entry:
    [isok,tt,uu,vv] = LpRmSmLm(x_F,y_F,phi_F);
    rmin = Rmin;
    x_F = Veh_x/rmin;
    y_F = Veh_y/rmin;Length=1000;
    phi_F = Veh_phi;type = 'NNNNN';
  state LmRpSpRp
    entry:
    [isok,tt,uu,vv] = LpRmSmRm(-x_F,y_F,-phi_F);
  state RpLmSmLm
    entry:
    [isok,tt,uu,vv] = LpRmSmRm(x_F,-y_F,-phi_F);
  state LpRmSmRm_main
    entry:
    [isok,tt,uu,vv] = LpRmSmRm(x_F,y_F,phi_F);
  state RmLpSpLp
    entry:
    [isok,tt,uu,vv] = LpRmSmRm(-x_F,-y_F,phi_F);
  state LmSmRmLp_main
    entry:
    xb = x_F*cos(phi_F)+y_F*sin(phi_F);
    yb = x_F*sin(phi_F)-y_F*cos(phi_F);
    [isok,tt,uu,vv] = LpRmSmLm(xb,yb ,phi_F);
  state LmRpSpLp
    entry:
    [isok,tt,uu,vv] = LpRmSmLm(-x_F,y_F,-phi_F);
  state RpLmSmRm
    entry:
    [isok,tt,uu,vv] = LpRmSmLm(x_F,-y_F,-phi_F);
  state RmLpSpRp
    entry:
    [isok,tt,uu,vv] = LpRmSmLm(-x_F,-y_F,phi_F);
  state RpSpRpLm
    entry:
    [isok,tt,uu,vv] = LpRmSmRm(-x_F,y_F,-phi_F);
  state LmSmLmRp
    entry:
    [isok,tt,uu,vv] = LpRmSmRm(x_F,-y_F,-phi_F);
  state RmSmRmLp_main
    entry:
    [isok,tt,uu,vv] = LpRmSmRm(x_F,y_F,phi_F);
  state LpSpLpRm
    entry:
    [isok,tt,uu,vv] = LpRmSmRm(-x_F,-y_F,phi_F);
    Length = 1000;m=0;n=0;
  state stand16
    Length = 1000;
    tt=0;vv=0;uu=0;
    n = 0;m= 0;
    type = 'NNNNN';
  state LpSpRpLm
    entry:
    [isok,tt,uu,vv] = LpRmSmLm(-xb,yb,-phi_F);
  state RmSmLmRp
    entry:
    [isok,tt,uu,vv] = LpRmSmLm(xb,-yb,-phi_F);
  state RpSpLpRm
    entry:
    [isok,tt,uu,vv] = LpRmSmLm(-x_F,-y_F,phi_F);
  state LpRmSmLm_ok
    Length = abs(tt) +abs(uu)+abs(vv);
    m = vv;vv=uu;uu=-pi/2;
    n = 0;
    type = 'LRSLN';
  state LmRpSpLp_ok
    Length = abs(tt) +abs(uu)+abs(vv);
    m = -vv;tt=-tt;vv=-uu;uu=-pi/2;
    n = 0;
    type = 'LRSLN';
  state RpLmSmRm_ok
    Length = abs(tt) +abs(uu)+abs(vv);
    m = vv;vv=uu;uu=-pi/2;
    n = 0;
    type = 'RLSRN';
  state RmLpSpRp_ok
    Length = abs(tt) +abs(uu)+abs(vv);
    m = -vv;tt=-tt;vv=-uu;uu=pi/2;
    n = 0;
    type = 'RLSRN';
  state LpRmSmRm_ok
    Length = abs(tt) +abs(uu)+abs(vv);
    m = -vv;tt=-tt;vv=-uu;uu=pi/2;
    n = 0;
    type = 'LRSRN';
  state LmRpSpRp_ok
    Length = abs(tt) +abs(uu)+abs(vv);
    m = -vv;tt=-tt;vv=-uu;uu=pi/2;
    n = 0;
    type = 'LRSRN';
  state RpLmSmLm_ok
    Length = abs(tt) +abs(uu)+abs(vv);
    m = vv; vv=uu;uu=-pi/2;
    n = 0;
    type = 'RLSLN';
  state RmLpSpLp_ok
    Length = abs(tt) +abs(uu)+abs(vv);
    m = -vv;tt=-tt;vv=-uu;uu=pi/2;
    n = 0;
    type = 'RLSLN';
  state LmSmRmLp_ok
    Length = abs(tt) +abs(uu)+abs(vv);
    m = tt;tt=vv;vv=-pi/2;
    n = 0;
    type = 'LRSLN';
  state LpSpRpLm_ok
    Length = abs(tt) +abs(uu)+abs(vv);
    m = -tt;tt=-vv;uu=-uu;vv=pi/2;
    n = 0;
    type = 'LSRLN';
  state RmSmLmRp_ok
    Length = abs(tt) +abs(uu)+abs(vv);
    m = tt;tt=vv;vv=-pi/2;
    n = 0;
    type = 'RSLRN';
  state RpSpLpRm_ok
    Length = abs(tt) +abs(uu)+abs(vv);
    m = -tt;tt=-vv;uu=-uu;vv=pi/2;
    n = 0;
    type = 'RSLRN';
  state RmSmRmLp_ok
    Length = abs(tt) +abs(uu)+abs(vv);
    m = tt;tt=vv;vv=-pi/2;
    n = 0;
    type = 'RSRLN';
  state RpSpRpLm_ok
    Length = abs(tt) +abs(uu)+abs(vv);
    m = -tt;tt=-vv;uu=-uu;vv=pi/2;
    n = 0;
    type = 'RSRLN';
  state LmSmLmRp_ok
    Length = abs(tt) +abs(uu)+abs(vv);
    m = tt;tt=vv;vv=-pi/2;
    n = 0;
    type = 'LSLRN';
  state LpSpLpRm_ok
    Length = abs(tt) +abs(uu)+abs(vv);
    m = -tt;tt=-vv;uu=-uu;vv=pi/2;
    n = 0;
    type = 'RSRLN';
  state stand
  state stand1
  state stand2
  state stand3
  state stand4
  state stand5
  state stand6
  state stand7
  state stand8
  state stand9
  state stand11
  state stand12
  state stand13
  state stand10
  state stand14
  state stand15
  (default) -> Begin
  LmRpSpRp -> RpLmSmLm [order 2] : [isok == 0]
  RpLmSmLm -> RmLpSpLp [order 2] : [isok == 0]
  LmRpSpLp -> RpLmSmRm [order 2] : [isok == 0]
  Begin -> LmRpSpLp [order 2] : [isok == 0]
  RpLmSmRm -> RmLpSpRp [order 1] : [isok == 0]
  RmLpSpLp -> LmSmRmLp_main [order 2] : [isok==0]
  LpRmSmRm_main -> LmRpSpRp [order 2] : [isok ==0]
  RmLpSpRp -> LpRmSmRm_main [order 1] : [isok == 0]
  RpSpRpLm -> LmSmLmRp [order 2] : [isok==0]
  Begin -> LpRmSmLm_ok [order 1] : [isok == 1]
  LmRpSpLp -> LmRpSpLp_ok [order 1] : [isok == 1]
  RpLmSmRm -> RpLmSmRm_ok [order 2] : [isok == 1]
  RmLpSpRp -> RmLpSpRp_ok [order 2] : [isok ==1]
  LpRmSmRm_main -> LpRmSmRm_ok [order 1] : [isok ==1]
  LmSmLmRp -> LpSpLpRm [order 2] : [isok == 0]
  LmRpSpRp -> LmRpSpRp_ok [order 1] : [isok ==1]
  RpLmSmLm -> RpLmSmLm_ok [order 1] : [isok ==1]
  LpSpRpLm -> RmSmLmRp [order 2] : [isok == 0]
  LmSmRmLp_main -> LpSpRpLm [order 2] : [isok == 0]
  RmSmLmRp -> RpSpLpRm [order 1] : [isok == 0]
  RmLpSpLp -> RmLpSpLp_ok [order 1] : [isok ==1]
  RmSmRmLp_main -> RpSpRpLm [order 2] : [isok ==0]
  RpSpLpRm -> RmSmRmLp_main [order 1] : [isok == 0]
  LpSpLpRm -> stand16 [order 2]
  LmSmRmLp_main -> LmSmRmLp_ok [order 1] : [isok == 1]
  LpSpRpLm -> LpSpRpLm_ok [order 1] : [isok == 1]
  RmSmLmRp -> RmSmLmRp_ok [order 2] : [isok == 1]
  RpSpLpRm -> RpSpLpRm_ok [order 2] : [isok ==1]
  RmSmRmLp_main -> RmSmRmLp_ok [order 1] : [isok ==1]
  RpSpRpLm -> RpSpRpLm_ok [order 1] : [isok ==1]
  LmSmLmRp -> LmSmLmRp_ok [order 1] : [isok ==1]
  LpSpLpRm -> LpSpLpRm_ok [order 1] : [isok ==1]
  LpRmSmLm_ok -> stand
  LmRpSpLp_ok -> stand1
  RpLmSmRm_ok -> stand2
  RmLpSpRp_ok -> stand3
  LpRmSmRm_ok -> stand4
  LmRpSpRp_ok -> stand5
  RpLmSmLm_ok -> stand6
  RmLpSpLp_ok -> stand7
  LmSmRmLp_ok -> stand8
  LpSpRpLm_ok -> stand9
  RmSmLmRp_ok -> stand10
  RpSpLpRm_ok -> stand11
  RmSmRmLp_ok -> stand12
  RpSpRpLm_ok -> stand13
  LmSmLmRp_ok -> stand14
  LpSpLpRm_ok -> stand15
  data: x function_input double; y function_input double; phi function_input double; isok function_output double; t function_output double; u function_output double; v function_output double; x function_input double; v function_output double; x function_input double; y function_input double; phi function_input double; isok function_output double; t function_output double; u function_output double; v function_output double; Veh_x input double; Veh_y input double; Veh_phi input double; Rmin input double; tt output double; uu output double; vv output double; m output double; n output double; Length output double; type output string; isok local double; phi_F local double; rmin local double; x_F local double; xb local double; y_F local double; yb local double; pi parameter
  function [isok,t,u,v] = LpRmSmRm(x,y,phi):
    | function [isok,t,u,v] = LpRmSmRm(x,y,phi)
    |     xi = x+sin(phi);
    |     eta = y-1-cos(phi);
    |     [theta,rho] = cart2pol(-eta,xi);
    |     if rho >= 2
    |         t = theta;
    |         u = 2-rho;
    |         v = mod2pi(t+pi/2-phi);
    |         if t >= 0 && u <= 0 && v <= 0
    |             isok = 1;
    |             return
    |         end
    |     end
    |     isok = 0;
    |     t = 0;
    |     u = 0;
    |     v = 0;
    | end
  function v = mod2pi(x):
    | function v = mod2pi(x)
    |     v = rem(x,2*pi);
    |     if v < -pi
    |         v = v+2*pi;
    |     elseif v > pi
    |         v = v-2*pi;
    |     end
    | end
  function [isok,t,u,v] = LpRmSmLm(x,y,phi):
    | function [isok,t,u,v] = LpRmSmLm(x,y,phi)
    |     xi = x-sin(phi);
    |     eta = y-1+cos(phi);
    |     [theta,rho] = cart2pol(xi,eta);
    |     if rho >= 2
    |         r = sqrt(rho^2-4);
    |         u = 2-r;
    |         t = mod2pi(theta+atan2(r,-2));
    |         v = mod2pi(phi-pi/2-t);
    |         if t >= 0 && u <= 0 && v <= 0
    |             isok = 1;
    |             return
    |         end
    |     end
    |     isok = 0;
    |     t = 0;
    |     u = 0;
    |     v = 0;
    | end

== stateflow chart TEST1231/FindRSheeps/RS/FindCCSCCPath ==
  state Begin
    entry:
    rmin = Rmin;
    x_F = Veh_x/rmin;
    y_F = Veh_y/rmin;Length=1000;
    phi_F = Veh_phi;type = 'NNNNN';
    [isok,tt,uu,vv] = LpRmSLmRp(x_F,y_F,phi_F);
  state stand4
    Length = 1000;
    tt=0;vv=0;uu=0;
    n = 0;m= 0;
    type = 'NNNNN';
  state LmRpSLpRm
    entry:
    [isok,tt,uu,vv] = LpRmSLmRp(-x_F,y_F,-phi_F);
  state RmLpSRpLm
    entry:
    [isok,tt,uu,vv] = LpRmSLmRp(x_F,-y_F,-phi_F);
  state RpLmSRmLp
    entry:
    [isok,tt,uu,vv] = LpRmSLmRp(-x_F,-y_F,phi_F);
    Length = 1000;m = 0;n = 0;
  state LmRpSLpRm_ok
    Length = abs(tt) +abs(uu)+abs(vv);
    tt=-tt;n = -vv;vv=-uu;m=pi/2;
    uu=pi/2;vv=uu;
    type = 'LRSLR';
  state LpRmSLmRp_ok
    Length = abs(tt) +abs(uu)+abs(vv);
    n = vv;vv=uu;m=-pi/2;
    uu=-pi/2;vv=uu;
    type = 'LRSLR';
  state RmLpSRpLm_ok
    Length = abs(tt) +abs(uu)+abs(vv);
    n = vv;vv=uu;m=-pi/2;
    uu=-pi/2;vv=uu;
    type = 'RLSRL';
  state RpLmSRmLp_ok
    Length = abs(tt) +abs(uu)+abs(vv);
    tt=-tt;n = -vv;vv=-uu;m=pi/2;
    uu=pi/2;vv=uu;
    type = 'RLSRL ';
  state stand
  state stand1
  state stand2
  state stand3
  (default) -> Begin
  LmRpSLpRm -> RmLpSRpLm [order 2] : [isok == 0]
  Begin -> LmRpSLpRm [order 2] : [isok == 0]
  RpLmSRmLp -> stand4 [order 2] : [isok==0]
  RmLpSRpLm -> RpLmSRmLp [order 1] : [isok == 0]
  Begin -> LpRmSLmRp_ok [order 1] : [isok == 1]
  LmRpSLpRm -> LmRpSLpRm_ok [order 1] : [isok == 1]
  RmLpSRpLm -> RmLpSRpLm_ok [order 2] : [isok == 1]
  RpLmSRmLp -> RpLmSRmLp_ok [order 1] : [isok ==1]
  LmRpSLpRm_ok -> stand1
  LpRmSLmRp_ok -> stand
  RmLpSRpLm_ok -> stand2
  RpLmSRmLp_ok -> stand3
  data: x function_input double; v function_output double; x function_input double; y function_input double; phi function_input double; isok function_output double; t function_output double; u function_output double; v function_output double; Veh_x input double; Veh_y input double; Veh_phi input double; Rmin input double; tt output double; uu output double; vv output double; m output double; n output double; Length output double; type output string; isok local double; phi_F local double; rmin local double; x_F local double; y_F local double; pi parameter
  function v = mod2pi(x):
    | function v = mod2pi(x)
    |     v = rem(x,2*pi);
    |     if v < -pi
    |         v = v+2*pi;
    |     elseif v > pi
    |         v = v-2*pi;
    |     end
    | end
  function [isok,t,u,v] = LpRmSLmRp(x,y,phi):
    | function [isok,t,u,v] = LpRmSLmRp(x,y,phi)
    |     xi = x+sin(phi);
    |     eta = y-1-cos(phi);
    |     [~,rho] = cart2pol(xi,eta);
    |     if rho >= 2
    |         u = 4-sqrt(rho^2-4);
    |         if u <= 0
    |             t = mod2pi(atan2((4-u)*xi-2*eta,-2*xi+(u-4)*eta));
    |             v = mod2pi(t-phi);
    |             if t >= 0 && v >= 0
    |                 isok = 1;
    |                 return
    |             end
    |         end
    |     end
    |     isok = 0;
    |     t = 0;
    |     u = 0;
    |     v = 0;
    | end
